simulink model "sampleModel1824"  (R2023a)
settings: Solver=VariableStepAuto  StartTime=0.0  StopTime=10.0  RelTol=1e-3
libraries: hdlsllib x6, simulink x1
settings Model: Creator=user1  LastModifiedBy=user1

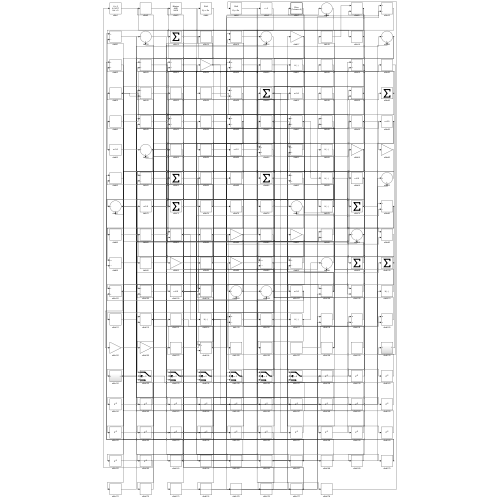
[thumbnail: Simulink's stored preview of the top-level diagram]
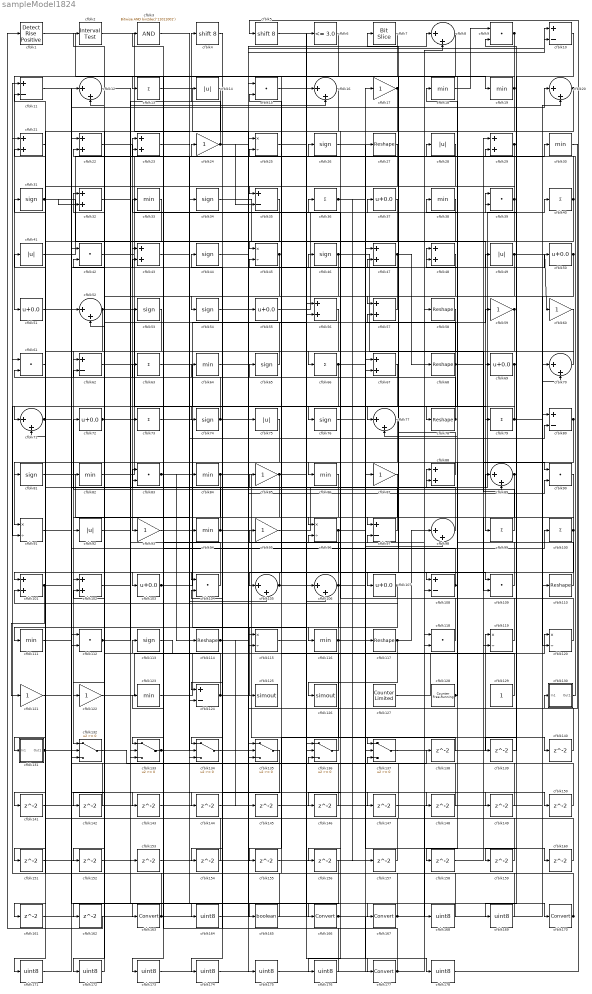
== system sampleModel1824 ==
  cfblk1 : hdlsllib/Logic and Bit Operations/Detect Rise Positive  vinit=0  OutDataTypeStr=boolean
  cfblk{10..11,35,62,80,97,108,124} (8 alike) : Sum  Inputs=+-
  cfblk{13,36,40,63,66,73,79,99..100} (9 alike) : Sum  Inputs=+
  cfblk{21..23,29,32,43,47..48,56..57,67,88,101..102} (14 alike) : Sum
  cfblk{37,50..51,55,69,72,103,107} (8 alike) : Bias  Bias=0.0  SaturateOnIntegerOverflow=off
  cfblk{9,15,39,42,61,83,90,104,109,112,118} (11 alike) : DotProduct  OutDataTypeStr=Inherit: Inherit via internal rule
  cfblk{8,12,16,20,52,70..71,77,89,98,105..106} (12 alike) : Sum  Inputs=|++
  cfblk{27,58,68,78,110,114,117} (7 alike) : Reshape
  cfblk{18..19,30,33,38,64,82,84,86,94,111,116,123} (13 alike) : MinMax
  cfblk{26,31,34,44,46,53..54,65,74,76,81,113} (12 alike) : Signum
  cfblk{25,45,91,96,115,119..120} (7 alike) : Product  Inputs=*/  RndMeth=Zero  SaturateOnIntegerOverflow=on
  cfblk{17,24,59..60,85,87,93,95,121..122} (10 alike) : Gain
  cfblk125 : ToWorkspace  VariableName=simout  SaveFormat=Timeseries  SampleTime=-1
  cfblk126 : ToWorkspace  VariableName=simout  SaveFormat=Timeseries  SampleTime=-1
  cfblk127 : hdlsllib/Sources/Counter Limited  uplimit=7  tsamp=-1
  cfblk128 : hdlsllib/Sources/Counter Free-Running  NumBits=16  tsamp=-1
  cfblk129 : Constant  SampleTime=-1
  cfblk130 : Subsystem
      settings: LibrarySourceBlock=|
      | hdlsllib/Ports &
      | Subsystems/Subsystem
  cfblk131 : Subsystem
      settings: LibrarySourceBlock=|
      | hdlsllib/Ports &
      | Subsystems/Subsystem
  cfblk{132..137} (6 alike) : Switch  SaturateOnIntegerOverflow=off  InputSameDT=off
  cfblk{138..162} (25 alike) : Delay  SampleTime=1
  cfblk{14,28,41,49,75,92} (6 alike) : Abs  SaturateOnIntegerOverflow=off
  cfblk{163,166..167,170,177} (5 alike) : DataTypeConversion  SaturateOnIntegerOverflow=off  RndMeth=Floor
  cfblk{164,168..169,171..176,178} (10 alike) : DataTypeConversion  OutDataTypeStr=uint8  SaturateOnIntegerOverflow=off  RndMeth=Floor
  cfblk165 : DataTypeConversion  OutDataTypeStr=boolean  SaturateOnIntegerOverflow=off  RndMeth=Floor
  cfblk2 : hdlsllib/Logic and Bit Operations/Interval Test  IntervalClosedRight=on  uplimit=0.5  IntervalClosedLeft=on  lowlimit=-0.5  OutDataTypeStr=boolean
  cfblk3 : simulink/Logic and Bit Operations/Bitwise Operator  logicop=AND  UseBitMask=on  BitMask=bin2dec('11011001')  BitMaskRealWorld=Stored Integer
      settings: LibrarySourceBlock=|
      | hdlsllib/Logic and Bit
      | Operations/Bitwise
      | Operator
  cfblk4 : ArithShift  BitShiftNumber=8
  cfblk5 : ArithShift  BitShiftNumber=8
  cfblk6 : hdlsllib/Logic and Bit Operations/Compare To Constant  relop=<=  const=3.0  OutDataTypeStr=boolean
  cfblk7 : hdlsllib/Logic and Bit Operations/Bit Slice  lidx=7  ridx=0
  wires:
  cfblk7/1 -> cfblk51/1
  cfblk83/1 -> cfblk114/1, cfblk165/1
  cfblk53/1 -> cfblk132/1
  cfblk113/1 -> cfblk120/1
  cfblk56/1 -> cfblk66/1
  cfblk35/1 -> cfblk45/1
  cfblk130/1(Out1) -> cfblk23/1
  cfblk47/1 -> cfblk68/1, cfblk57/1
  cfblk27/1 -> cfblk126/1
  cfblk3/1 -> cfblk166/1
  cfblk99/1 -> cfblk72/1
  cfblk21/1 -> cfblk111/1
  cfblk41/1 -> cfblk24/1
  cfblk61/1 -> cfblk31/1
  cfblk120/1 -> cfblk36/1
  cfblk34/1 -> cfblk99/1
  cfblk106/1 -> cfblk96/2, cfblk160/1, cfblk171/1
  cfblk19/1 -> cfblk86/1, cfblk13/1
  cfblk82/1 -> cfblk37/1
  cfblk25/1 -> cfblk106/1
  cfblk57/1 -> cfblk54/1
  cfblk20/1 -> cfblk122/1, cfblk43/1
  cfblk100/1 -> cfblk92/1, cfblk146/1
  cfblk36/1 -> cfblk67/1, cfblk157/1
  cfblk17/1 -> cfblk97/1, cfblk96/1
  cfblk89/1 -> cfblk39/1, cfblk134/3
  cfblk49/1 -> cfblk60/1, cfblk164/1
  cfblk22/1 -> cfblk93/1
  cfblk88/1 -> cfblk45/2
  cfblk98/1 -> cfblk41/1
  cfblk85/1 -> cfblk134/1, cfblk39/2
  cfblk55/1 -> cfblk27/1
  cfblk86/1 -> cfblk133/1
  cfblk18/1 -> cfblk9/1
  cfblk48/1 -> cfblk103/1
  cfblk84/1 -> cfblk137/1, cfblk162/1
  cfblk6/1 -> cfblk163/1
  cfblk127/1 -> cfblk110/1
  cfblk45/1 -> cfblk53/1, cfblk142/1
  cfblk119/1 -> cfblk95/1
  cfblk94/1 -> cfblk10/1, cfblk63/1
  cfblk134/1 -> cfblk55/1
  cfblk123/1 -> cfblk29/1
  cfblk5/1 -> cfblk177/1
  cfblk44/1 -> cfblk109/1
  cfblk73/1 -> cfblk136/1
  cfblk95/1 -> cfblk40/1
  cfblk133/1 -> cfblk105/2, cfblk147/1
  cfblk42/1 -> cfblk26/1
  cfblk110/1 -> cfblk48/1
  cfblk104/1 -> cfblk83/1
  cfblk116/1 -> cfblk28/1, cfblk62/2, cfblk155/1
  cfblk72/1 -> cfblk17/1, cfblk50/1
  cfblk63/1 -> cfblk79/1
  cfblk112/1 -> cfblk97/2, cfblk14/1
  cfblk23/1 -> cfblk34/1
  cfblk80/1 -> cfblk124/1, cfblk158/1
  cfblk67/1 -> cfblk116/1
  cfblk1/1 -> cfblk56/1
  cfblk74/1 -> cfblk8/1, cfblk61/2
  cfblk52/1 -> cfblk77/1, cfblk134/2, cfblk151/1
  cfblk103/1 -> cfblk16/1, cfblk58/1, cfblk30/1, cfblk80/2
  cfblk118/1 -> cfblk33/1
  cfblk68/1 -> cfblk32/1, cfblk90/1, cfblk104/1, cfblk133/3
  cfblk2/1 -> cfblk84/1
  cfblk26/1 -> cfblk108/1
  cfblk77/1 -> cfblk91/1
  cfblk97/1 -> cfblk44/1
  cfblk108/1 -> cfblk18/1, cfblk23/2, cfblk57/2
  cfblk105/1 -> cfblk101/1, cfblk150/1
  cfblk30/1 -> cfblk130/1(In1)
  cfblk33/1 -> cfblk62/1
  cfblk114/1 -> cfblk90/2, cfblk29/2, cfblk145/1
  cfblk107/1 -> cfblk125/1, cfblk101/2
  cfblk62/1 -> cfblk49/1
  cfblk79/1 -> cfblk76/1, cfblk70/2
  cfblk14/1 -> cfblk71/1
  cfblk92/1 -> cfblk16/2
  cfblk109/1 -> cfblk77/2
  cfblk90/1 -> cfblk109/2
  cfblk101/1 -> cfblk121/1, cfblk43/2
  cfblk59/1 -> cfblk73/1, cfblk102/1
  cfblk81/1 -> cfblk124/2
  cfblk12/1 -> cfblk170/1
  cfblk16/1 -> cfblk132/2
  cfblk115/1 -> cfblk88/1
  cfblk29/1 -> cfblk131/1(In1), cfblk169/1
  cfblk129/1 -> cfblk85/1
  cfblk9/1 -> cfblk78/1, cfblk107/1
  cfblk38/1 -> cfblk74/1
  cfblk124/1 -> cfblk115/1, cfblk52/2
  cfblk39/1 -> cfblk82/1, cfblk35/1
  cfblk15/1 -> cfblk19/1
  cfblk8/1 -> cfblk105/1
  cfblk137/1 -> cfblk119/1
  cfblk70/1 -> cfblk69/1
  cfblk11/1 -> cfblk167/1
  cfblk122/1 -> cfblk94/1
  cfblk69/1 -> cfblk112/2, cfblk159/1
  cfblk54/1 -> cfblk46/1
  cfblk60/1 -> cfblk81/1
  cfblk65/1 -> cfblk42/2
  cfblk111/1 -> cfblk20/1
  cfblk66/1 -> cfblk59/1, cfblk91/2
  cfblk128/1 -> cfblk38/1, cfblk48/2
  cfblk96/1 -> cfblk98/2, cfblk161/1
  cfblk93/1 -> cfblk25/2
  cfblk71/1 -> cfblk47/2, cfblk143/1
  cfblk58/1 -> cfblk71/2
  cfblk78/1 -> cfblk2/1, cfblk7/1
  cfblk136/1 -> cfblk65/1
  cfblk50/1 -> cfblk120/2, cfblk133/2
  cfblk131/1(Out1) -> cfblk88/2, cfblk100/1
  cfblk13/1 -> cfblk135/2
  cfblk51/1 -> cfblk52/1
  cfblk31/1 -> cfblk117/1, cfblk32/2
  cfblk91/1 -> cfblk89/1
  cfblk24/1 -> cfblk4/1, cfblk10/2, cfblk35/2
  cfblk40/1 -> cfblk132/3, cfblk22/2
  cfblk46/1 -> cfblk89/2, cfblk115/2
  cfblk117/1 -> cfblk98/1, cfblk176/1
  cfblk132/1 -> cfblk138/1
  cfblk138/1 -> cfblk136/2
  cfblk10/1 -> cfblk139/1
  cfblk139/1 -> cfblk9/2
  cfblk76/1 -> cfblk140/1
  cfblk140/1 -> cfblk25/1
  cfblk37/1 -> cfblk141/1
  cfblk141/1 -> cfblk20/2
  cfblk142/1 -> cfblk112/1
  cfblk143/1 -> cfblk108/2
  cfblk32/1 -> cfblk144/1
  cfblk144/1 -> cfblk56/2
  cfblk145/1 -> cfblk70/1
  cfblk146/1 -> cfblk104/2
  cfblk121/1 -> cfblk148/1
  cfblk148/1 -> cfblk47/1
  cfblk43/1 -> cfblk149/1
  cfblk149/1 -> cfblk42/1
  cfblk150/1 -> cfblk136/3
  cfblk151/1 -> cfblk135/3
  cfblk75/1 -> cfblk152/1
  cfblk152/1 -> cfblk135/1
  cfblk102/1 -> cfblk153/1
  cfblk153/1 -> cfblk106/2
  cfblk4/1 -> cfblk154/1
  cfblk154/1 -> cfblk21/2
  cfblk155/1 -> cfblk67/2
  cfblk28/1 -> cfblk156/1
  cfblk157/1 -> cfblk83/2
  cfblk158/1 -> cfblk119/2
  cfblk159/1 -> cfblk137/3
  cfblk160/1 -> cfblk22/1
  cfblk161/1 -> cfblk137/2
  cfblk162/1 -> cfblk1/1
  cfblk163/1 -> cfblk102/2, cfblk75/1
  cfblk164/1 -> cfblk6/1
  cfblk165/1 -> cfblk3/1
  cfblk166/1 -> cfblk80/1, cfblk8/2, cfblk178/1
  cfblk167/1 -> cfblk61/1, cfblk15/1
  cfblk147/1 -> cfblk168/1
  cfblk168/1 -> cfblk11/1
  cfblk169/1 -> cfblk11/2
  cfblk170/1 -> cfblk15/2, cfblk21/1
  cfblk171/1 -> cfblk12/1
  cfblk156/1 -> cfblk172/1
  cfblk172/1 -> cfblk12/2
  cfblk87/1 -> cfblk173/1
  cfblk173/1 -> cfblk118/2
  cfblk135/1 -> cfblk174/1
  cfblk174/1 -> cfblk87/1
  cfblk64/1 -> cfblk175/1
  cfblk175/1 -> cfblk118/1
  cfblk176/1 -> cfblk64/1
  cfblk177/1 -> cfblk123/1, cfblk113/1
  cfblk178/1 -> cfblk5/1

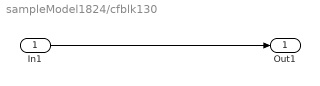
== system sampleModel1824/cfblk130 ==
  In1 : Inport
  Out1 : Outport
  wires:
  In1/1 -> Out1/1

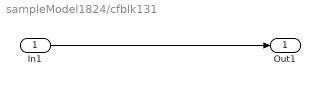
== system sampleModel1824/cfblk131 ==
  In1 : Inport
  Out1 : Outport
  wires:
  In1/1 -> Out1/1
